simulink model "video_viewer"  (R2023b)
settings: Solver=VariableStepAuto  StartTime=0.0  StopTime=10.0  RelTol=1e-3
undefined symbols (not defined in the file or in its folder): none, Rec, SDTV, videoinput
libraries: visionconversions x2, imaqlib x1, dspstat3 x1
settings Model: Creator=Bread  LastModifiedBy=Bread

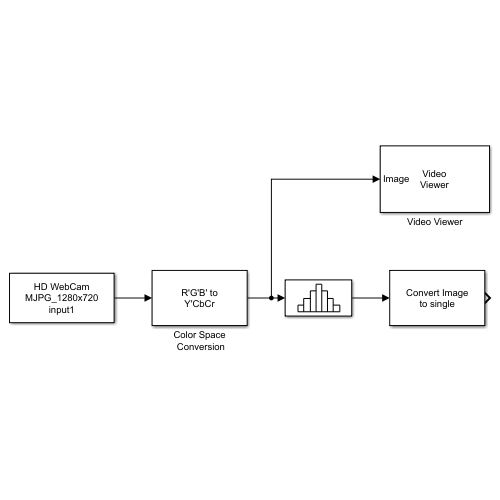
[thumbnail: Simulink's stored preview of the top-level diagram]
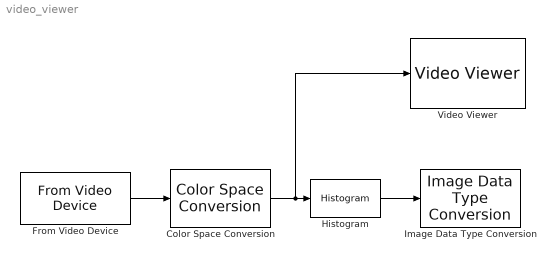
== system video_viewer ==
  Color Space Conversion : visionconversions/Color Space  Conversion  conversion=Obsolete  conversionActive=R'G'B' to Y'CbCr  wp_str=D65  rec=Rec. 601 (SDTV)  sys=1125/60/2:1  imagePorts=One multidimensional signal
  From Video Device : imaqlib/From Video Device  DeviceMenu=winvideo 1 (HD WebCam)  Device=winvideo 1 (HD WebCam)  ObjConstructor=videoinput('winvideo', 1)  VideoFormatMenu=MJPG_1280x720  VideoFormat=MJPG_1280x720  VideoSource=input1  ROIPosition=[0 0 720 1280]  EnableHWTrigger=off  TriggerConfiguration=none/none  SampleTime=1/30  OutputPortsMode=One multidimensional signal  DataType=single  CanDoHWTrigger=no  ReturnedColorSpace=rgb  BlockHandle=4.0002  ROIWidth=1280  ROIHeight=720  ROIColumn=0  ROIRow=0  EngXMLPath=C:\Program Files\MATLAB\R2023b\toolbox\imaq\imaq\private  DevXMLPath=C:\ProgramData\MATLAB\SupportPackages\R2023b\toolbox\imaq\supportpackages\genericvideo\adaptor\win64  EngLibPath=C:\Program Files\MATLAB\R2023b\toolbox\imaq\imaqblks\imaqmex\win64  ColorSpace=rgb  BayerSensorAlignment=grbg  ImaqMode=off
  Histogram : dspstat3/Histogram  umin=0  umax=10  nbins=11  operateOver=Each column  Dimension=1  normalized=off  run=off  reset=on  trigtype=Non-zero sample  colComp=on  roundingMode=Floor  overflowMode=off
  Image Data Type Conversion : visionconversions/Image Data Type Conversion  outDT=single  isSigned=on  wordLen=16  numFracBits=0
  Video Viewer : VideoViewer  FigPos=[474 535 418 304]
  wires:
  Color Space Conversion/1 -> Video Viewer/1, Histogram/1
  From Video Device/1 -> Color Space Conversion/1
  Histogram/1 -> Image Data Type Conversion/1
